simulink model "sldemo_dblcart1"  (R2022a)
settings: Solver=ode23  StartTime=0  StopTime=40  MaxStep=0.1  RelTol=1e-3  AbsTol=1e-6
PostLoadFcn:
  | crtanim2([],[],[],0,1);
model workspace (MAT data in the model file):
  ka = 1
  m1 = 1
  m2 = 1
Description:
  | Double Spring Mass System
  | 
  | This example shows how to model a double spring-mass-damper system with a periodically
  | varying forcing function.  Associated with the example is an animation function
  | that will automatically open a figure window and display to it. In this system,
  | the only sensor is attached to the mass on the left, and the actuator is
  | attached to the mass on the left. State estimation and LQR control are used.
settings Model: PacingRate=2.500000  Creator=The MathWorks, Inc.  LastModifiedBy=whatastarrynight
settings SolverCC: AutoScaleAbsTol=off  AlgebraicLoopSolver=TrustRegion
settings DataIOCC: ExternalInput=[]  InitialState=[]  SaveFormat=Array  SaveOutput=off  SaveTime=off
settings OptimizationCC: BlockReduction=off  BooleanDataType=off  InitFltsAndDblsToZero=on  LifeSpan=inf  BufferReusableBoundary=off
settings DebuggingCC: SaveWithParameterizedLinksMsg=none  UnderspecifiedInitializationDetection=Classic  MergeDetectMultiDrivingBlocksExec=none  SignalResolutionControl=TryResolveAllWithWarning  MultiTaskDSMMsg=warning  MultiTaskCondExecSysMsg=none  FcnCallInpInsideContextMsg=warning  UnconnectedInputMsg=warning  UnconnectedOutputMsg=warning  UnconnectedLineMsg=warning  BusObjectLabelMismatch=none  SFUnexpectedBacktrackingDiag=warning  SFNoUnconditionalDefaultTransitionDiag=warning  SFExecutionAtInitializationDiag=none  SFMachineParentedDataDiag=warning  ArithmeticOperatorsInVariantConditions=warning
settings HardwareCC: ProdBitPerPointer=32  ProdBitPerSizeT=32  ProdBitPerPtrDiffT=32  ProdLargestAtomicFloat=None  ProdIntDivRoundTo=Undefined  ProdEndianess=Unspecified  ProdWordSize=32  ProdHWDeviceType=32-bit Generic  TargetUnknown=on
settings ModelReferenceCC: PropagateSignalLabelsOutOfModel=off
settings SFSimCC: SimUseLocalCustomCode=off  CustomCodeUndefinedFunction=UseInterfaceOnly
settings RTWCC: Description=Generic Real-Time Target  RTWUseLocalCustomCode=off
settings CodeAppCC: StateflowObjectComments=on
settings GRTTargetCC: TargetFcnLib=ansi_tfl_tmw.mat  TargetLangStandard=C89/C90 (ANSI)  CombineOutputUpdateFcns=off  GRTInterface=on
settings ConfigComp: CovMetricSettings=dw  CovSaveCumulativeToWorkspaceVar=on  CovSaveSingleToWorkspaceVar=on  CovExternalEMLEnable=off

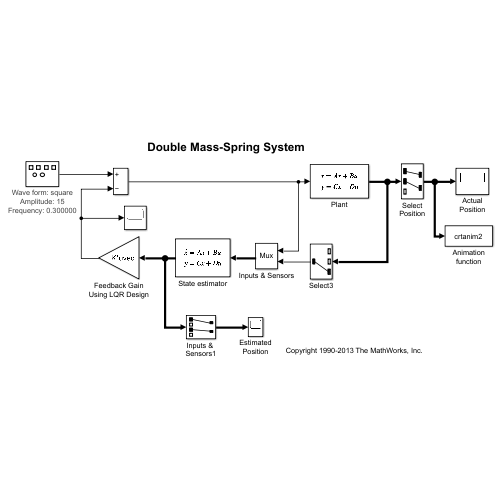
[thumbnail: Simulink's stored preview of the top-level diagram]
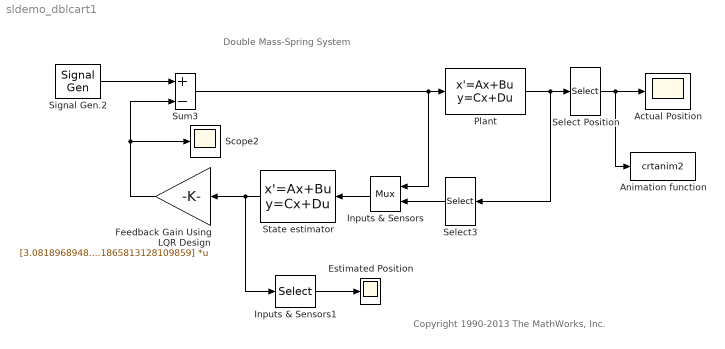
== system sldemo_dblcart1 ==
  note: Double Mass-Spring System
  note: Copyright 1990-2013 The MathWorks, Inc.
  Actual Position : Scope
  Animation function : S-Function  FunctionName=crtanim2  Parameters=0.1  SFunctionDeploymentMode=off  EnableBusSupport=off
      settings: DeleteFcn=shh = get(0,'ShowHiddenHandles');set(0,'ShowHiddenHandles','on');if ~isempty(findobj('type','figure','name','dblcart1 Animation'));close('dblcart1 Animation'); end;set(0,'ShowHiddenHandles',shh);
  Estimated Position : Scope
  Feedback Gain Using LQR Design : Gain  Gain=[3.0818968948757903 2.4826988922846818 0.0803807652925895 3.1865813128109859]  Multiplication=Matrix(K*u) (u vector)
  Inputs & Sensors1 : Selector  InputPortWidth=4  IndexOptions=Index vector (dialog)  Indices=[1 3]  OutputSizes=1
  Inputs & Sensors : Mux  Inputs=2
  Plant : StateSpace  A=[0 1 0 0; -ka/m1 0 ka/m1 0; 0 0 0 1;ka/m2 0 -ka/m2 0]  B=[0; 1; 0; 0]  C=[1 0 0 0;0 0 1 0;0 0 1 0]  D=zeros(3,1)  InitialCondition=0
  Scope2 : Scope
  Select Position : Selector  InputPortWidth=3  IndexOptions=Index vector (dialog)  Indices=[1,2]  OutputSizes=1
  Select3 : Selector  InputPortWidth=3  IndexOptions=Index vector (dialog)  Indices=3  OutputSizes=1
  Signal Gen.2 : SignalGenerator  WaveForm=square  Amplitude=15  Frequency=0.300000  Units=rad/sec
      settings: AttributesFormatString=|
      | Wave form: %<WaveForm>
      | Amplitude: %<Amplitude>
      | Frequency: %<Frequency>
  State estimator : StateSpace  A=[0 1 -31.450729701314597 0;-1 0 44.853668760256895 0;0 0 -46.659940598124535 1;1 0 -89.575028310252492 0]  B=[0 31.450729701314597;1 -43.853668760256895;0 46.659940598124535;0 88.575028310252492]  C=[1 0 0 0;0 1 0 0;0 0 1 0;0 0 0 1]  D=[0 0;0 0;0 0;0 0]  InitialCondition=0
  Sum3 : Sum  Inputs=+-  InputSameDT=on  SaturateOnIntegerOverflow=on  OutDataTypeStr=Inherit: Same as first input
  wires:
  State estimator/1 -> Inputs & Sensors1/1, Feedback Gain Using LQR Design/1
  Inputs & Sensors/1 -> State estimator/1
  Sum3/1 -> Plant/1, Inputs & Sensors/1
  Feedback Gain Using LQR Design/1 -> Scope2/1, Sum3/2
  Plant/1 -> Select3/1, Select Position/1
  Signal Gen.2/1 -> Sum3/1
  Inputs & Sensors1/1 -> Estimated Position/1
  Select3/1 -> Inputs & Sensors/2
  Select Position/1 -> Animation function/1, Actual Position/1
